simulink model "AOO"  (R2022a)
settings: Solver=FixedStepAuto  StartTime=0.0  StopTime=10.0  FixedStep=1e-3  RelTol=1e-3  EnableMultiTasking=on
undefined symbols (not defined in the file): D10, D11, D2, D4, D5, D8, PTA0, PTA2, PTB23, PTB9, PTD0, PTD2
libraries: frdmk64flib x6
settings Model: ExtModeTrigDuration=5  Creator=kemij  LastModifiedBy=bmile
settings OptimizationCC: EnhancedBackFolding=on  PassReuseOutputArgsAs=Individual arguments  ZeroExternalMemoryAtStartup=off  ZeroInternalMemoryAtStartup=off  MaxStackSize=64  OptimizeBlockOrder=speed  DifferentSizesBufferReuse=on  OptimizationCustomize=off  EfficientTunableParamExpr=on
settings DebuggingCC: ParameterTunabilityLossMsg=error
settings HardwareCC: ProdBitPerPointer=32  ProdBitPerSizeT=32  ProdBitPerPtrDiffT=32  ProdLargestAtomicInteger=Long  ProdLargestAtomicFloat=Double  ProdWordSize=32  ProdHWDeviceType=ARM Compatible->ARM Cortex
settings SFSimCC: MATLABDynamicMemAlloc=off
settings RTWCC: SystemTargetFile=ert.tlc  HardwareBoard=NXP FRDM-K64F  TLCOptions="-aInlineSetEventsForThisBaseRateFcn=TLC_FALSE -aSuppressMultiTaskScheduler=TLC_FALSE  -aRateBasedStepFcn=0"  TemplateMakefile=ert_default_tmf  Toolchain=GNU Tools for ARM Embedded Processors
settings CodeAppCC: ForceParamTrailComments=on  IgnoreCustomStorageClasses=off  OperatorAnnotations=on  SimulinkDataObjDesc=on  SFDataObjDesc=on  InsertBlockDesc=on
settings ERTTargetCC: ExtModeTransport=4  ExtModeMexFile=sendToCommService

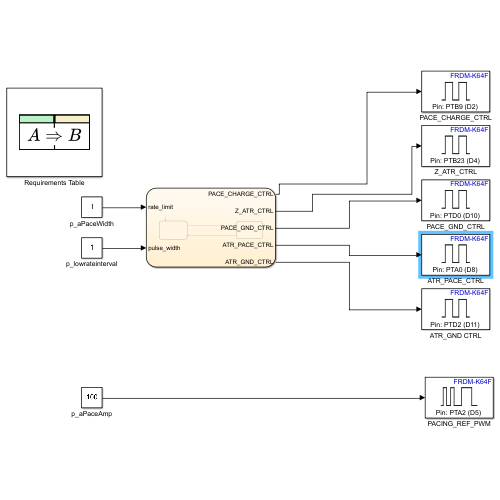
[thumbnail: Simulink's stored preview of the top-level diagram]
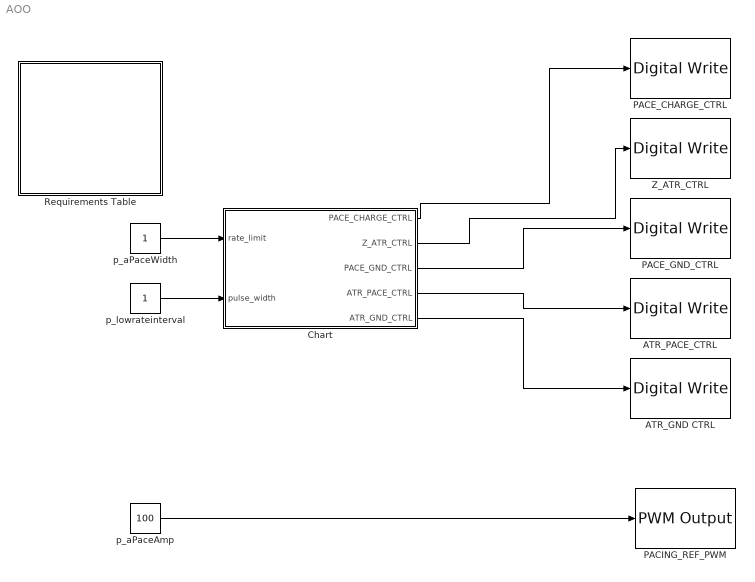
== system AOO ==
  ATR_GND CTRL : frdmk64flib/Digital Write  Whichpin=PTD2 (D11)
  ATR_PACE_CTRL : frdmk64flib/Digital Write  Whichpin=PTA0 (D8)
  Chart : Stateflow chart  TreatAsAtomicUnit=on
  PACE_CHARGE_CTRL : frdmk64flib/Digital Write  Whichpin=PTB9 (D2)
  PACE_GND_CTRL : frdmk64flib/Digital Write  Whichpin=PTD0 (D10)
  PACING_REF_PWM : frdmk64flib/PWM Output  Whichpin=PTA2 (D5)  InitialFrequency=2000  InitialDutyCycle=0
  Requirements Table : Requirements Table  TreatAsAtomicUnit=on
  Z_ATR_CTRL : frdmk64flib/Digital Write  Whichpin=PTB23 (D4)
  p_aPaceAmp : Constant  Value=100
  p_aPaceWidth : Constant
  p_lowrateinterval : Constant
  wires:
  p_aPaceWidth/1 -> Chart/1(rate_limit)
  p_lowrateinterval/1 -> Chart/2(pulse_width)
  p_aPaceAmp/1 -> PACING_REF_PWM/1
  Chart/5(ATR_GND_CTRL) -> ATR_GND CTRL/1
  Chart/4(ATR_PACE_CTRL) -> ATR_PACE_CTRL/1
  Chart/3(PACE_GND_CTRL) -> PACE_GND_CTRL/1
  Chart/2(Z_ATR_CTRL) -> Z_ATR_CTRL/1
  Chart/1(PACE_CHARGE_CTRL) -> PACE_CHARGE_CTRL/1

== stateflow chart AOO/Chart ==
  state Charging_Discharging
    entry:
    ATR_PACE_CTRL = false
    PACE_CHARGE_CTRL = true
    ATR_GND_CTRL = true
    PACE_GND_CTRL = true
    Z_ATR_CTRL=false
  state Pace_Heart
    entry:
    ATR_PACE_CTRL = true
    PACE_CHARGE_CTRL = false
    PACE_GND_CTRL = true
    ATR_GND_CTRL = false
  (default) -> Charging_Discharging
  Charging_Discharging -> Pace_Heart : after(((1/rate_limit)*60000)-pulse_width,msec)
  Pace_Heart -> Charging_Discharging : after(pulse_width,msec)
  data: rate_limit input; pulse_width input; PACE_CHARGE_CTRL output boolean; Z_ATR_CTRL output boolean; PACE_GND_CTRL output boolean; ATR_PACE_CTRL output boolean; ATR_GND_CTRL output boolean

== stateflow chart AOO/Requirements Table ==
  (default) -> (junction 1073741860)
  (junction 1073741860) -> (junction 1073741861) : {
      | % SF_REQ_REV_07
      | }
  (junction 1073741861) -> (junction 1073741863) : {
      | % HEADER_ASSIGNMENTS
      |
      | }
  (junction 1073741863) -> (junction 1073741865) : {
      | % START_A_4
      | }
  (junction 1073741865) -> (junction 1073741867) : {
      | }
  (junction 1073741867) -> (junction 1073741869)
  (junction 1073741869) -> (junction 1073741871) : {
      | }
  (junction 1073741871) -> (junction 1073741873) : {
      | % END_A_4
      | }
  (junction 1073741873) -> (junction 1073741898) : {
      | % START_R_1
      | }
  (junction 1073741898) -> (junction 1073741900) : {
      | }
  (junction 1073741900) -> (junction 1073741902) : {
      |
      |
      | }
  (junction 1073741902) -> (junction 1073741904) : {
      | }
  (junction 1073741904) -> (junction 1073741906) : {
      | % END_R_1
      | }
